simulink model "PB2M_001_007_RL"  (R2024a)
settings: Solver=FixedStepDiscrete  StartTime=0.0  StopTime=inf  FixedStep=[global_ST]  RelTol=1e-3
model workspace (MAT data in the model file):
  Var = 0
values from neighbouring files (symbols this model uses):
  global_ST = 1    [SimControl_v3_rl.m]    (also in SimControl_v4.m)
  global_time = [0:1:8784]'    [SimControl_v3_rl.m]    (also in SimControl_v4.m)
undefined symbols (not defined in the file or in its folder): acc, AEL, allActions, AMB, ATR, Bttry, CGH2, CGO2, CHP, COMPR, contActSpace, Ctrl, DiscIntNeverNeededParam, DIST, DRY, GASF, Gasf, imit_action_noise_variance, lowerLim, MES, NumEpisodes, NumImitLearning, numtraineps, PV, th, upperLim, vanilla, WT
libraries: simulink x1, rllib x1
(part 1 of 2)
settings Model: Creator=hogrebe  LastModifiedBy=salomon_p
settings SolverCC: AlgebraicLoopSolver=TrustRegion
settings DataIOCC: SaveOutput=off  DSMLogging=off  InspectSignalLogs=on  SaveTime=off
settings OptimizationCC: BlockReduction=off
settings DebuggingCC: SignalInfNanChecking=error  UnconnectedInputMsg=warning  UnconnectedOutputMsg=warning  UnconnectedLineMsg=warning
settings ModelReferenceCC: EnableRefExpFcnMdlSchedulingChecks=on
settings RTWCC: GPUComputeCapability=3.5  DLArmComputeVersion=19.05

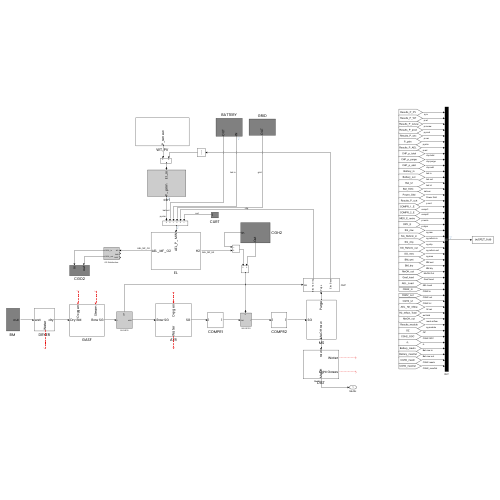
[thumbnail: Simulink's stored preview of the top-level diagram]
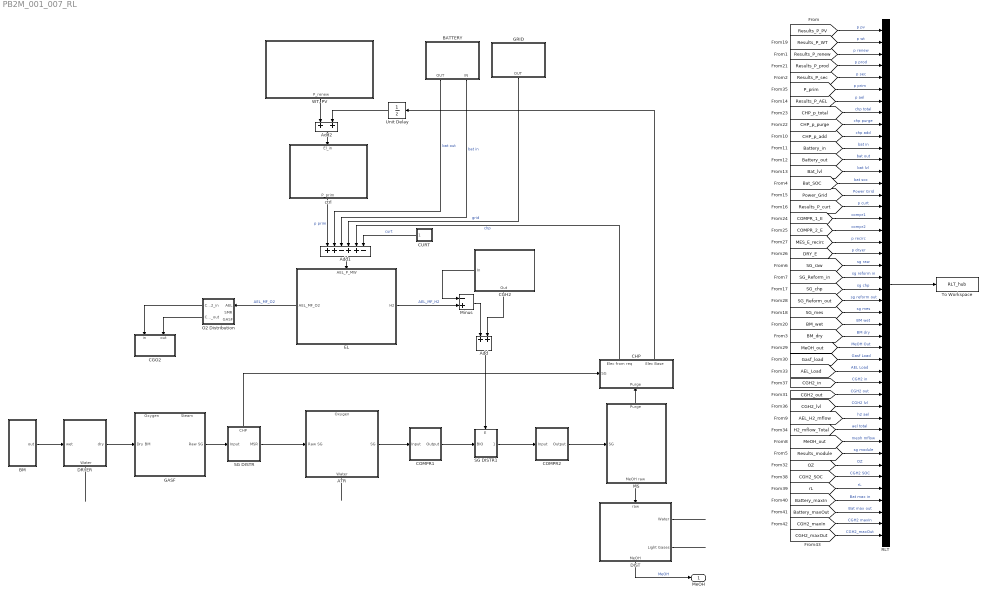
== system PB2M_001_007_RL ==
  ATR : Subsystem
      settings: PortSchema="{\"entries\":[{\"content\":{\"sides\":[{\"content\":{\"connectorIds\":[\"In1\"]},\"type\":\"ConnectorPlacement.EquallySpacedRectSide\",\"uuid\":\"d95d7370-a768-4e71-99c5-23d50f67aabe\"},{\"content\":{\"connectorIds\":[\"Out1\"],\"side\":\"RIGHT\"},\"type\":\"ConnectorPlacement.EquallySpacedRectSide\",\"uuid\":\"3437d418-ce7d-423d-8668-067a2caa5d39\"},{\"content\":{\"connectorIds\":[\"In2\"],\"side\":\"TOP\"},\"type\":\"ConnectorPlacement.EquallySpacedRectSide\",\"uuid\":\"c8aa7c63-1393-4bbc-8660-d82006d9d42e\"},{\"content\":{\"connectorIds\":[\"Out2\"],\"side\":\"BOTTOM\"},\"type\":\"ConnectorPlacement.EquallySpacedRectSide\",\"uuid\":\"8d079498-92c7-4ac5-81b3-d100ec68b2bd\"}]},\"type\":\"ConnectorPlacement.EquallySpacedConnector\",\"uuid\":\"07712eec-a256-4c23-80e6-026550a38bce\"}],\"packageUris\":[\"http://schema.mathworks.com/mf0/Connector/R2020b\"],\"version\":\"1.0\"}"
  Add : Sum
  Add1 : Sum  Inputs=++-++-
  Add2 : Sum
  BATTERY : Subsystem
      settings: PortSchema="{\"entries\":[{\"content\":{\"sides\":[{\"content\":{},\"type\":\"ConnectorPlacement.EquallySpacedRectSide\",\"uuid\":\"b156ae25-26b3-4eee-ac7f-e302bdaac2ab\"},{\"content\":{\"side\":\"RIGHT\"},\"type\":\"ConnectorPlacement.EquallySpacedRectSide\",\"uuid\":\"f3a3b929-51c5-4419-b41e-ec6279a18565\"},{\"content\":{\"side\":\"TOP\"},\"type\":\"ConnectorPlacement.EquallySpacedRectSide\",\"uuid\":\"01f6443f-63f0-4718-804f-9bad3a04ddfb\"},{\"content\":{\"connectorIds\":[\"Out1\",\"Out2\"],\"side\":\"BOTTOM\"},\"type\":\"ConnectorPlacement.EquallySpacedRectSide\",\"uuid\":\"cbf48387-64e5-4e53-bde3-6e14dbb130f7\"}]},\"type\":\"ConnectorPlacement.EquallySpacedConnector\",\"uuid\":\"4aa34124-3e08-49a0-9db9-a8367ba9f9e9\"}],\"packageUris\":[\"http://schema.mathworks.com/mf0/Connector/R2020b\"],\"version\":\"1.0\"}"
  "BM " : Subsystem
      settings: PortSchema="{\"entries\":[{\"content\":{\"sides\":[{\"content\":{},\"type\":\"ConnectorPlacement.EquallySpacedRectSide\",\"uuid\":\"b6854826-029a-462c-abc7-1ad3a9c8d91d\"},{\"content\":{\"side\":\"RIGHT\"},\"type\":\"ConnectorPlacement.EquallySpacedRectSide\",\"uuid\":\"c18fafb4-eebd-4b53-a025-0d4bc890a5f2\"},{\"content\":{\"connectorIds\":[\"Out1\"],\"side\":\"TOP\"},\"type\":\"ConnectorPlacement.EquallySpacedRectSide\",\"uuid\":\"39a115de-f541-49b1-95b5-0fdea67e1df4\"}]},\"type\":\"ConnectorPlacement.EquallySpacedConnector\",\"uuid\":\"d3505c7c-2ca5-40d6-998f-e51c69df56d8\"}],\"packageUris\":[\"http://schema.mathworks.com/mf0/Connector/R2020b\"],\"version\":\"1.0\"}"
  CGH2 : Subsystem
      settings: PortSchema="{\"entries\":[{\"content\":{\"sides\":[{\"content\":{\"connectorIds\":[\"Out2\"]},\"type\":\"ConnectorPlacement.EquallySpacedRectSide\",\"uuid\":\"c54b6fc4-3adc-4d22-bd7c-d1fb71d09cc2\"},{\"content\":{\"side\":\"RIGHT\"},\"type\":\"ConnectorPlacement.EquallySpacedRectSide\",\"uuid\":\"cb46d28f-124e-4362-a527-4ffafd6ca6aa\"},{\"content\":{\"side\":\"TOP\"},\"type\":\"ConnectorPlacement.EquallySpacedRectSide\",\"uuid\":\"cd2bfd56-c3bb-4b21-97bf-19e28abe6737\"},{\"content\":{\"connectorIds\":[\"Out1\"],\"side\":\"BOTTOM\"},\"type\":\"ConnectorPlacement.EquallySpacedRectSide\",\"uuid\":\"e393c782-34b5-435a-9a6b-fea68a5f76b1\"}]},\"type\":\"ConnectorPlacement.EquallySpacedConnector\",\"uuid\":\"04f91959-6cb0-408d-b188-ebba459e7bf2\"}],\"packageUris\":[\"http://schema.mathworks.com/mf0/Connector/R2020b\"],\"version\":\"1.0\"}"
  CGO2 : Subsystem
      settings: PortSchema="{\"entries\":[{\"content\":{\"sides\":[{\"content\":{},\"type\":\"ConnectorPlacement.EquallySpacedRectSide\",\"uuid\":\"5fd0e465-b758-40c5-99c0-bd502cf80220\"},{\"content\":{\"side\":\"RIGHT\"},\"type\":\"ConnectorPlacement.EquallySpacedRectSide\",\"uuid\":\"8c2bf71d-dd8a-4c38-9726-2100ecfb4157\"},{\"content\":{\"connectorIds\":[\"In1\",\"In2\"],\"side\":\"TOP\"},\"type\":\"ConnectorPlacement.EquallySpacedRectSide\",\"uuid\":\"9b00925e-eb9b-456e-968f-5d87047a8706\"}]},\"type\":\"ConnectorPlacement.EquallySpacedConnector\",\"uuid\":\"2f6cfec4-9fe2-41ff-9b0f-2d3a7383541d\"}],\"packageUris\":[\"http://schema.mathworks.com/mf0/Connector/R2020b\"],\"version\":\"1.0\"}"
  CHP : Subsystem
      settings: PortSchema="{\"entries\":[{\"content\":{\"sides\":[{\"content\":{\"connectorIds\":[\"In1\"]},\"type\":\"ConnectorPlacement.EquallySpacedRectSide\",\"uuid\":\"455e4cb2-b7ce-40b3-9267-45576cb92a35\"},{\"content\":{\"side\":\"RIGHT\"},\"type\":\"ConnectorPlacement.EquallySpacedRectSide\",\"uuid\":\"26266506-6e66-4bc0-bccd-a9e779dcae16\"},{\"content\":{\"connectorIds\":[\"Out1\",\"Out2\"],\"side\":\"TOP\"},\"type\":\"ConnectorPlacement.EquallySpacedRectSide\",\"uuid\":\"0bfe460e-97a8-4cdd-8918-1c56f22f3fbd\"},{\"content\":{\"connectorIds\":[\"In2\"],\"side\":\"BOTTOM\"},\"type\":\"ConnectorPlacement.EquallySpacedRectSide\",\"uuid\":\"d15a681e-1531-4d34-b913-d07bfab7e09a\"}]},\"type\":\"ConnectorPlacement.EquallySpacedConnector\",\"uuid\":\"864e4265-4fc9-4c94-8dd3-96a5c52575a2\"}],\"packageUris\":[\"http://schema.mathworks.com/mf0/Connector/R2020b\"],\"version\":\"1.0\"}"
  COMPR1 : Subsystem
  COMPR2 : Subsystem
  CURT : Subsystem
      settings: PortSchema="{\"entries\":[{\"content\":{\"sides\":[{\"content\":{\"connectorIds\":[\"Out1\"]},\"type\":\"ConnectorPlacement.EquallySpacedRectSide\",\"uuid\":\"455e4cb2-b7ce-40b3-9267-45576cb92a35\"},{\"content\":{\"side\":\"RIGHT\"},\"type\":\"ConnectorPlacement.EquallySpacedRectSide\",\"uuid\":\"26266506-6e66-4bc0-bccd-a9e779dcae16\"},{\"content\":{\"side\":\"TOP\"},\"type\":\"ConnectorPlacement.EquallySpacedRectSide\",\"uuid\":\"0bfe460e-97a8-4cdd-8918-1c56f22f3fbd\"}]},\"type\":\"ConnectorPlacement.EquallySpacedConnector\",\"uuid\":\"864e4265-4fc9-4c94-8dd3-96a5c52575a2\"}],\"packageUris\":[\"http://schema.mathworks.com/mf0/Connector/R2020b\"],\"version\":\"1.0\"}"
  DIST : Subsystem
      settings: PortSchema="{\"entries\":[{\"content\":{\"sides\":[{\"content\":{},\"type\":\"ConnectorPlacement.EquallySpacedRectSide\",\"uuid\":\"9bb20e76-c8c0-4ce3-bfa2-fd978c659bcc\"},{\"content\":{\"connectorIds\":[\"Out1\",\"Out2\"],\"side\":\"RIGHT\"},\"type\":\"ConnectorPlacement.EquallySpacedRectSide\",\"uuid\":\"12d31df4-77c9-4a5c-9a6c-fd7c89038c05\"},{\"content\":{\"connectorIds\":[\"In1\"],\"side\":\"TOP\"},\"type\":\"ConnectorPlacement.EquallySpacedRectSide\",\"uuid\":\"3a96496e-8d88-4b7f-91f0-6f8e8152b6d3\"},{\"content\":{\"connectorIds\":[\"Out3\"],\"side\":\"BOTTOM\"},\"type\":\"ConnectorPlacement.EquallySpacedRectSide\",\"uuid\":\"4bc833e2-fc0a-44a4-bcf0-3ebf0863e835\"}]},\"type\":\"ConnectorPlacement.EquallySpacedConnector\",\"uuid\":\"bb9c8f09-08c9-4a34-bdc9-5c844495fddc\"}],\"packageUris\":[\"http://schema.mathworks.com/mf0/Connector/R2020b\"],\"version\":\"1.0\"}"
  DRYER : Subsystem
      settings: PortSchema="{\"entries\":[{\"content\":{\"sides\":[{\"content\":{},\"type\":\"ConnectorPlacement.EquallySpacedRectSide\",\"uuid\":\"4ebfcccc-776f-4872-9d0b-9643b5960bad\"},{\"content\":{\"connectorIds\":[\"Out1\"],\"side\":\"RIGHT\"},\"type\":\"ConnectorPlacement.EquallySpacedRectSide\",\"uuid\":\"52af1a20-21ba-42da-ac0d-5cc3ed928415\"},{\"content\":{\"connectorIds\":[\"Out2\"],\"side\":\"TOP\"},\"type\":\"ConnectorPlacement.EquallySpacedRectSide\",\"uuid\":\"35b3f618-6f56-49d4-89a8-2314405479bc\"},{\"content\":{\"connectorIds\":[\"In1\"],\"side\":\"BOTTOM\"},\"type\":\"ConnectorPlacement.EquallySpacedRectSide\",\"uuid\":\"a7ad5d18-a31c-4405-a5bd-3fe59bb19813\"}]},\"type\":\"ConnectorPlacement.EquallySpacedConnector\",\"uuid\":\"90f717a7-269d-4abb-8032-a33661c35212\"}],\"packageUris\":[\"http://schema.mathworks.com/mf0/Connector/R2020b\"],\"version\":\"1.0\"}"
  EL : Subsystem
      settings: PortSchema="{\"entries\":[{\"content\":{\"sides\":[{\"content\":{\"connectorIds\":[\"Out2\"]},\"type\":\"ConnectorPlacement.EquallySpacedRectSide\",\"uuid\":\"e86b81d9-d45f-45ad-8c80-2ef5c9159145\"},{\"content\":{\"connectorIds\":[\"Out1\"],\"side\":\"RIGHT\"},\"type\":\"ConnectorPlacement.EquallySpacedRectSide\",\"uuid\":\"b091bd34-fe91-455d-8135-92fc1e1b5bd7\"},{\"content\":{\"connectorIds\":[\"In1\"],\"side\":\"TOP\"},\"type\":\"ConnectorPlacement.EquallySpacedRectSide\",\"uuid\":\"804c6318-ad33-4a07-b17e-e0d2fd6b4b2f\"}]},\"type\":\"ConnectorPlacement.EquallySpacedConnector\",\"uuid\":\"e581105a-7c66-468d-8489-1abddd5a4bb6\"}],\"packageUris\":[\"http://schema.mathworks.com/mf0/Connector/R2020b\"],\"version\":\"1.0\"}"
  GASF : Subsystem
      settings: PortSchema="{\"entries\":[{\"content\":{\"sides\":[{\"content\":{\"connectorIds\":[\"In1\"]},\"type\":\"ConnectorPlacement.EquallySpacedRectSide\",\"uuid\":\"5e6aa46e-d817-493b-8b8b-abb4dd1f40ec\"},{\"content\":{\"connectorIds\":[\"Out1\"],\"side\":\"RIGHT\"},\"type\":\"ConnectorPlacement.EquallySpacedRectSide\",\"uuid\":\"1936bb9e-e226-4528-9325-ecfa0f913ec2\"},{\"content\":{\"connectorIds\":[\"In2\",\"In3\"],\"side\":\"TOP\"},\"type\":\"ConnectorPlacement.EquallySpacedRectSide\",\"uuid\":\"7345e236-0dce-483e-9dbc-f4ebd743c5fa\"}]},\"type\":\"ConnectorPlacement.EquallySpacedConnector\",\"uuid\":\"c88779f2-c803-4e9a-bd9c-ad3f8fae613a\"}],\"packageUris\":[\"http://schema.mathworks.com/mf0/Connector/R2020b\"],\"version\":\"1.0\"}"
  GRID : Subsystem
      settings: PortSchema="{\"entries\":[{\"content\":{\"sides\":[{\"content\":{},\"type\":\"ConnectorPlacement.EquallySpacedRectSide\",\"uuid\":\"13ddf689-c473-4fae-8488-05ba2c53be01\"},{\"content\":{\"side\":\"RIGHT\"},\"type\":\"ConnectorPlacement.EquallySpacedRectSide\",\"uuid\":\"3edd6540-09f8-47a0-8af0-925a1a207bbe\"},{\"content\":{\"side\":\"TOP\"},\"type\":\"ConnectorPlacement.EquallySpacedRectSide\",\"uuid\":\"e7e0af70-0c4e-4701-890f-2bc2f1b60263\"},{\"content\":{\"connectorIds\":[\"Out1\"],\"side\":\"BOTTOM\"},\"type\":\"ConnectorPlacement.EquallySpacedRectSide\",\"uuid\":\"aae9c7fc-ae1b-458f-888e-dcbddd5e368f\"}]},\"type\":\"ConnectorPlacement.EquallySpacedConnector\",\"uuid\":\"9fa59c12-9be8-49ba-a862-8cdac5f592f4\"}],\"packageUris\":[\"http://schema.mathworks.com/mf0/Connector/R2020b\"],\"version\":\"1.0\"}"
  MS : Subsystem
      settings: PortSchema="{\"entries\":[{\"content\":{\"sides\":[{\"content\":{\"connectorIds\":[\"In1\"]},\"type\":\"ConnectorPlacement.EquallySpacedRectSide\",\"uuid\":\"7c68cb95-e770-413e-a40e-672fd8604812\"},{\"content\":{\"side\":\"RIGHT\"},\"type\":\"ConnectorPlacement.EquallySpacedRectSide\",\"uuid\":\"6240a65a-2dbc-4a6e-817e-2ab31946396e\"},{\"content\":{\"connectorIds\":[\"Out2\"],\"side\":\"TOP\"},\"type\":\"ConnectorPlacement.EquallySpacedRectSide\",\"uuid\":\"1a1b519e-0693-45b9-a906-950b0dca57a1\"},{\"content\":{\"connectorIds\":[\"Out1\"],\"side\":\"BOTTOM\"},\"type\":\"ConnectorPlacement.EquallySpacedRectSide\",\"uuid\":\"e87dd805-e630-4a2f-8388-2c51cd14fe9e\"}]},\"type\":\"ConnectorPlacement.EquallySpacedConnector\",\"uuid\":\"e16e5d91-de04-48fc-b44b-fdb042a92f84\"}],\"packageUris\":[\"http://schema.mathworks.com/mf0/Connector/R2020b\"],\"version\":\"1.0\"}"
  Minus : Sum  Inputs=-+
  O2 Distribution : Subsystem
      settings: PortSchema="{\"entries\":[{\"content\":{\"sides\":[{\"content\":{\"connectorIds\":[\"Out3\",\"Out4\"]},\"type\":\"ConnectorPlacement.EquallySpacedRectSide\",\"uuid\":\"30156f9c-db5e-4257-aeed-83f2c1c2e5bf\"},{\"content\":{\"connectorIds\":[\"In1\",\"Out1\",\"Out2\"],\"side\":\"RIGHT\"},\"type\":\"ConnectorPlacement.EquallySpacedRectSide\",\"uuid\":\"c3a4c4df-5b27-475f-87a9-b45da9a3b436\"},{\"content\":{\"side\":\"TOP\"},\"type\":\"ConnectorPlacement.EquallySpacedRectSide\",\"uuid\":\"5997053d-e240-46ef-b6d7-4f9a3a1c0d15\"}]},\"type\":\"ConnectorPlacement.EquallySpacedConnector\",\"uuid\":\"10d495fb-251b-444d-bd0a-f6bbcb16daf1\"}],\"packageUris\":[\"http://schema.mathworks.com/mf0/Connector/R2020b\"],\"version\":\"1.0\"}"
  RLT : BusCreator  Inputs=44
  SG DISTR : Subsystem
      settings: PortSchema="{\"entries\":[{\"content\":{\"sides\":[{\"content\":{},\"type\":\"ConnectorPlacement.EquallySpacedRectSide\",\"uuid\":\"e86b81d9-d45f-45ad-8c80-2ef5c9159145\"},{\"content\":{\"connectorIds\":[\"Out1\"],\"side\":\"RIGHT\"},\"type\":\"ConnectorPlacement.EquallySpacedRectSide\",\"uuid\":\"b091bd34-fe91-455d-8135-92fc1e1b5bd7\"},{\"content\":{\"connectorIds\":[\"In1\"],\"side\":\"TOP\"},\"type\":\"ConnectorPlacement.EquallySpacedRectSide\",\"uuid\":\"804c6318-ad33-4a07-b17e-e0d2fd6b4b2f\"},{\"content\":{\"connectorIds\":[\"Out2\"],\"side\":\"BOTTOM\"},\"type\":\"ConnectorPlacement.EquallySpacedRectSide\",\"uuid\":\"fb2b571c-70ad-41c0-9018-552f5e98e285\"}]},\"type\":\"ConnectorPlacement.EquallySpacedConnector\",\"uuid\":\"e581105a-7c66-468d-8489-1abddd5a4bb6\"}],\"packageUris\":[\"http://schema.mathworks.com/mf0/Connector/R2020b\"],\"version\":\"1.0\"}"
  SG DISTR1 : Subsystem
      settings: PortSchema="{\"entries\":[{\"content\":{\"sides\":[{\"content\":{},\"type\":\"ConnectorPlacement.EquallySpacedRectSide\",\"uuid\":\"e9c91cab-8c69-4152-b789-7325d2e32e4b\"},{\"content\":{\"connectorIds\":[\"In2\"],\"side\":\"RIGHT\"},\"type\":\"ConnectorPlacement.EquallySpacedRectSide\",\"uuid\":\"b801369b-5c93-4438-bd90-0992b326086c\"},{\"content\":{\"connectorIds\":[\"In1\"],\"side\":\"TOP\"},\"type\":\"ConnectorPlacement.EquallySpacedRectSide\",\"uuid\":\"e103e961-9a42-4e45-906c-e9068e5e276c\"},{\"content\":{\"connectorIds\":[\"Out1\"],\"side\":\"BOTTOM\"},\"type\":\"ConnectorPlacement.EquallySpacedRectSide\",\"uuid\":\"0e96afff-5922-401c-b36e-06eb0842909a\"}]},\"type\":\"ConnectorPlacement.EquallySpacedConnector\",\"uuid\":\"2ea93f77-6b27-4245-9c93-a72fb1fe7fa6\"}],\"packageUris\":[\"http://schema.mathworks.com/mf0/Connector/R2020b\"],\"version\":\"1.0\"}"
  To Workspace : ToWorkspace  VariableName=RLT_hub  SampleTime=-1
  Unit Delay : UnitDelay  SampleTime=-1  HasFrameUpgradeWarning=on
  "WT, PV" : Subsystem
      settings: PortSchema="{\"entries\":[{\"content\":{\"sides\":[{\"content\":{},\"type\":\"ConnectorPlacement.EquallySpacedRectSide\",\"uuid\":\"8a2d1ae0-dccb-4b14-8547-5eeedb1731af\"},{\"content\":{\"side\":\"RIGHT\"},\"type\":\"ConnectorPlacement.EquallySpacedRectSide\",\"uuid\":\"3fb157a2-f839-4f36-8a45-db822d022818\"},{\"content\":{\"side\":\"TOP\"},\"type\":\"ConnectorPlacement.EquallySpacedRectSide\",\"uuid\":\"528eda02-61b1-46fc-814d-d4347d4497c7\"},{\"content\":{\"connectorIds\":[\"Out1\"],\"side\":\"BOTTOM\"},\"type\":\"ConnectorPlacement.EquallySpacedRectSide\",\"uuid\":\"9515b46c-adb3-49ca-b783-afbfd8bcb61a\"}]},\"type\":\"ConnectorPlacement.EquallySpacedConnector\",\"uuid\":\"11973188-1db2-4f1c-be62-25a3f427210a\"}],\"packageUris\":[\"http://schema.mathworks.com/mf0/Connector/R2020b\"],\"version\":\"1.0\"}"
  ctrl : Subsystem
      settings: PortSchema="{\"entries\":[{\"content\":{\"sides\":[{\"content\":{},\"type\":\"ConnectorPlacement.EquallySpacedRectSide\",\"uuid\":\"29211eeb-3776-4ac1-8b6e-260e730243bf\"},{\"content\":{\"side\":\"RIGHT\"},\"type\":\"ConnectorPlacement.EquallySpacedRectSide\",\"uuid\":\"53fb8f12-056e-46ec-aa17-61752852cd78\"},{\"content\":{\"connectorIds\":[\"In1\"],\"side\":\"TOP\"},\"type\":\"ConnectorPlacement.EquallySpacedRectSide\",\"uuid\":\"01e66cb5-7d7a-44e4-93db-ae92dadb6fda\"},{\"content\":{\"connectorIds\":[\"Out1\"],\"side\":\"BOTTOM\"},\"type\":\"ConnectorPlacement.EquallySpacedRectSide\",\"uuid\":\"c79a4ef3-496c-4d69-ab69-9c29ac94c10a\"}]},\"type\":\"ConnectorPlacement.EquallySpacedConnector\",\"uuid\":\"562cb731-47de-4bfb-9a4e-cc780a8c656b\"}],\"packageUris\":[\"http://schema.mathworks.com/mf0/Connector/R2020b\"],\"version\":\"1.0\"}"
  MeOH : Outport
  wires:
  EL/2(AEL_MF_O2) -> O2 Distribution/1(AEL)  "AEL_MF_O2"
  O2 Distribution/4(CGO2_out) -> CGO2/2(out)
  O2 Distribution/3(CGO2_in) -> CGO2/1(in)
  SG DISTR/2(MSR) -> ATR/1(Raw SG)
  DRYER/2(dry) -> GASF/1(Dry BM)
  GASF/1(Raw SG) -> SG DISTR/1(Input)
  ATR/1(SG) -> COMPR1/1(Input)
  SG DISTR1/1(Output) -> COMPR2/1(Input)
  SG DISTR/1(CHP) -> CHP/1(SG)
  "BM "/1(out) -> DRYER/1(wet)
  COMPR2/1(Output) -> MS/1(SG)
  ctrl/1(P_prim) -> Add1/1  "p prim"
  Add1/1 -> EL/1(AEL_P_MW)
  CHP/1(Elec from req) -> Add1/5  "chp"
  BATTERY/1(OUT) -> Add1/2  "bat out"
  BATTERY/2(IN) -> Add1/3  "bat in"
  GRID/1(OUT) -> Add1/4  "grid"
  CURT/1(Output) -> Add1/6  "curt"
  COMPR1/1(Output) -> SG DISTR1/1(BIO)
  RLT/1 -> To Workspace/1
  [SG_raw] -> RLT/21  "sg raw"
  [COMPR_2_E] -> RLT/18  "compr2"
  [Results_P_PV] -> RLT/1  "p pv"
  [Results_P_renew] -> RLT/3  "p renew"
  [Results_P_curt] -> RLT/16  "p curt"
  [Battery_in] -> RLT/11  "bat in"
  [Power_Grid] -> RLT/15  "Power Grid"
  [Bat_SOC] -> RLT/14  "bat soc"
  [CHP_p_purge] -> RLT/9  "chp purge"
  [Results_P_AEL] -> RLT/7  "p ael"
  [P_prim] -> RLT/6  "p prim"
  [CHP_p_total] -> RLT/8  "chp total"
  [COMPR_1_E] -> RLT/17  "compr1"
  [Results_P_sec] -> RLT/5  "p sec"
  [MES_E_recirc] -> RLT/19  "p recirc"
  MS/2(Purge) -> CHP/2(Purge)
  Add2/1 -> ctrl/1(El_in)
  "WT, PV"/1(P_renew) -> Add2/1
  DRYER/1(Water) -> ?
  ATR/2(Water) -> ?
  MS/1(MeOH raw) -> DIST/1(raw)
  DIST/3(MeOH) -> MeOH/1  "MeOH"
  DIST/1(Water) -> ?
  DIST/2(Light Gases) -> ?
  [SG_Reform_in] -> RLT/22  "sg reform in"
  [Results_P_prod] -> RLT/4  "p prod"
  [Battery_out] -> RLT/12  "bat out"
  [Bat_lvl] -> RLT/13  "bat lvl"
  [Results_P_WT] -> RLT/2  "p wt"
  ? -> GASF/3(Steam)
  ? -> GASF/2(Oxygen)
  ? -> ATR/2(Oxygen)
  [SG_Reform_out] -> RLT/24  "sg reform out"
  [SG_mes] -> RLT/25  "sg mes"
  [BM_wet] -> RLT/26  "BM wet"
  [BM_dry] -> RLT/27  "BM dry"
  [MeOH_out] -> RLT/28  "MeOH Out"
  CHP/2(Elec Base) -> Unit Delay/1
  Unit Delay/1 -> Add2/2
  CGH2/1(Out) -> Add/2
  [Gasf_load] -> RLT/29  "Gasf Load"
  [CGH2_in] -> RLT/31  "CGH2 in"
  EL/1(H2) -> Minus/2  "AEL_MF_H2"
  Minus/1 -> Add/1
  CGH2/2(In) -> Minus/1
  [H2_mflow_Total] -> RLT/35  "ael total"
  [CHP_p_add] -> RLT/10  "chp add"
  [SG_chp] -> RLT/23  "sg chp"
  [DRY_E] -> RLT/20  "p dryer"
  [AEL_Load] -> RLT/30  "AEL Load"
  [CGH2_out] -> RLT/32  "CGH2 out"
  [CGH2_lvl] -> RLT/33  "CGH2 lvl"
  [AEL_H2_mflow] -> RLT/34  "h2 ael"
  [MeOH_out] -> RLT/36  "meoh mflow"
  [Results_module] -> RLT/37  "sg module"
  [OZ] -> RLT/38  "OZ"
  Add/1 -> SG DISTR1/2(E)
  [CGH2_SOC] -> RLT/39  "CGH2 SOC"
  [rL] -> RLT/40  "rL"
  [Battery_maxIn] -> RLT/41  "Bat max in"
  [Battery_maxOut] -> RLT/42  "Bat max out"
  [CGH2_maxIn] -> RLT/43  "CGH2 maxIn"
  [CGH2_maxOut] -> RLT/44  "CGH2_maxOut"

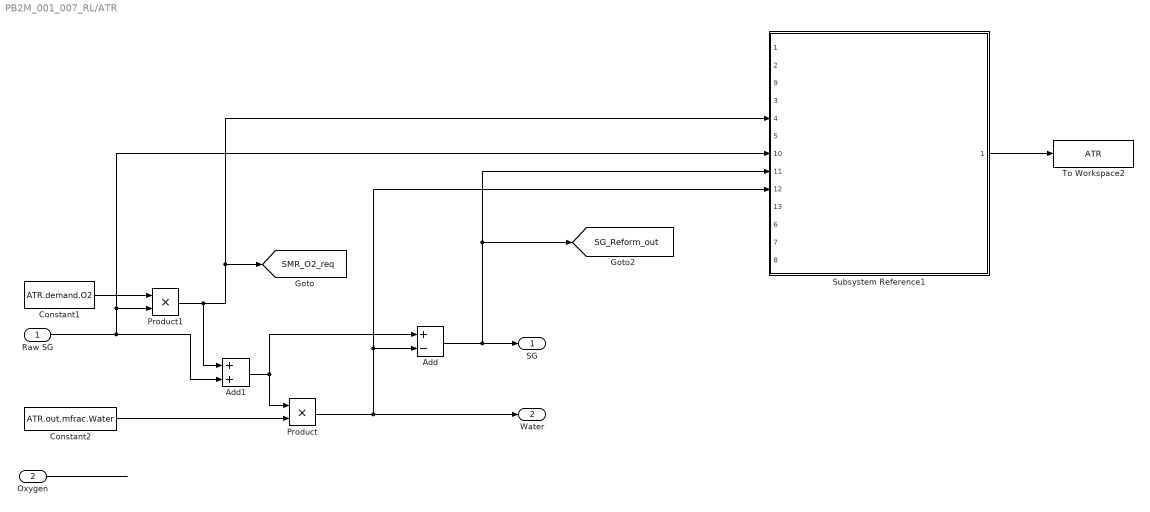
== system PB2M_001_007_RL/ATR ==
  Raw SG : Inport
  Oxygen : Inport  Port=2
  Add : Sum  Inputs=+-
  Add1 : Sum
  Constant1 : Constant  Value=ATR.demand.O2
  Constant2 : Constant  Value=ATR.out.mfrac.Water
  Product : Product
  Product1 : Product
  Subsystem Reference1 : Subsystem  ReferencedSubsystem=PB2M_RltHub_002
      settings: PortSchema="{\"entries\":[{\"content\":{\"sides\":[{\"content\":{\"connectorIds\":[\"In1\",\"In2\",\"In9\",\"In3\",\"In4\",\"In5\",\"In10\",\"In11\",\"In12\",\"In13\",\"In6\",\"In7\",\"In8\"]},\"type\":\"ConnectorPlacement.EquallySpacedRectSide\",\"uuid\":\"c0facf1f-1082-4e5e-a2dc-e6e5892eaa43\"},{\"content\":{\"connectorIds\":[\"Out1\"],\"side\":\"RIGHT\"},\"type\":\"ConnectorPlacement.EquallySpacedRectSide\",\"uuid\":\"0b7dd7b0-e6ba-4d46-903a-281e0aa5a817\"},{\"content\":{\"side\":\"TOP\"},\"type\":\"ConnectorPlacement.EquallySpacedRectSide\",\"uuid\":\"7e96b7db-a9f3-428f-bb56-8b966044c518\"}]},\"type\":\"ConnectorPlacement.EquallySpacedConnector\",\"uuid\":\"c0112396-a54d-4537-ae03-3d933c26b43e\"}],\"packageUris\":[\"http://schema.mathworks.com/mf0/Connector/R2020b\"],\"version\":\"1.0\"}"
  To Workspace2 : ToWorkspace  VariableName=ATR  SampleTime=-1
  SG : Outport
  Water : Outport  Port=2
  tag scope: SG_Reform_out=global, SMR_O2_req=global
  wires:
  Product1/1 -> [SMR_O2_req], Subsystem Reference1/4, Add1/1
  Raw SG/1 -> Product1/2, Subsystem Reference1/10, Add1/2
  Constant2/1 -> Product/2
  Product/1 -> Water/1, Subsystem Reference1/12, Add/2
  Add/1 -> [SG_Reform_out], Subsystem Reference1/11, SG/1
  Oxygen/1 -> ?
  Subsystem Reference1/1 -> To Workspace2/1
  Constant1/1 -> Product1/1
  Add1/1 -> Add/1, Product/1

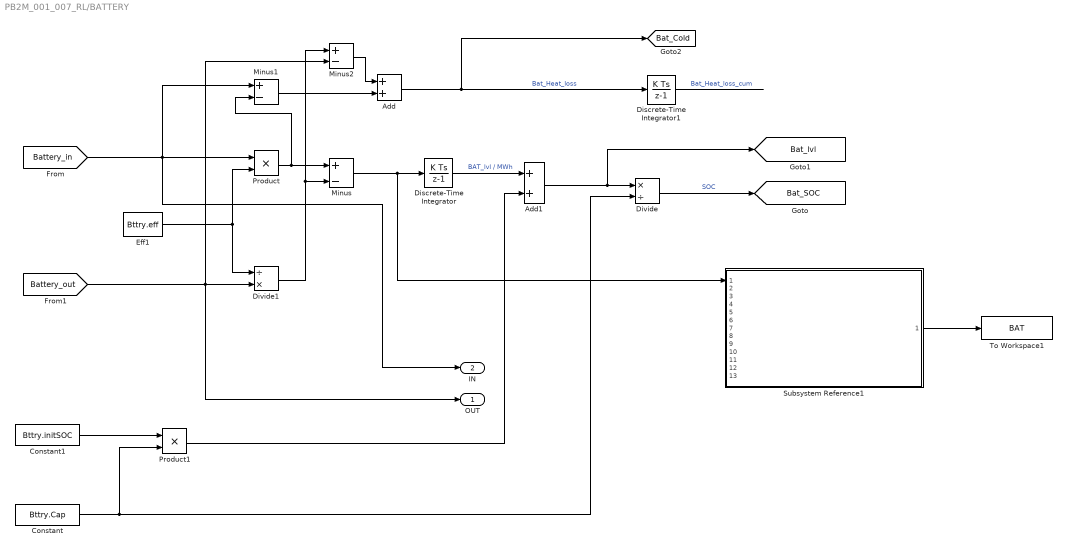
== system PB2M_001_007_RL/BATTERY ==
  Add : Sum
  Add1 : Sum
  Constant : Constant  Value=Bttry.Cap
  Constant1 : Constant  Value=Bttry.initSOC
  Discrete-Time Integrator : DiscreteIntegrator  SampleTime=-1  ICPrevOutput=DiscIntNeverNeededParam  ICPrevScaledInput=DiscIntNeverNeededParam
  Discrete-Time Integrator1 : DiscreteIntegrator  SampleTime=-1  ICPrevOutput=DiscIntNeverNeededParam  ICPrevScaledInput=DiscIntNeverNeededParam
  Divide : Product  Inputs=*/
  Divide1 : Product  Inputs=/*
  Eff1 : Constant  Value=Bttry.eff
  Minus : Sum  Inputs=+-
  Minus1 : Sum  Inputs=+-
  Minus2 : Sum  Inputs=+-
  Product : Product
  Product1 : Product
  Subsystem Reference1 : Subsystem  ReferencedSubsystem=PB2M_RltHub_002
  To Workspace1 : ToWorkspace  VariableName=BAT  SampleTime=-1
  OUT : Outport
  IN : Outport  Port=2
  tag scope: Bat_Cold=global, Bat_SOC=global, Bat_lvl=global
  wires:
  Constant/1 -> Divide/2, Product1/2
  Divide/1 -> [Bat_SOC]  "SOC"
  Product/1 -> Minus1/2, Minus/1
  Divide1/1 -> Minus2/1, Minus/2
  Eff1/1 -> Divide1/1, Product/2
  Minus1/1 -> Add/2
  Minus2/1 -> Add/1
  Add/1 -> [Bat_Cold], Discrete-Time Integrator1/1  "Bat_Heat_loss"
  Discrete-Time Integrator1/1 -> ?  "Bat_Heat_loss_cum"
  [Battery_out] -> Divide1/2, OUT/1, Minus2/2
  [Battery_in] -> IN/1, Minus1/1, Product/1
  Minus/1 -> Subsystem Reference1/1, Discrete-Time Integrator/1
  Add1/1 -> [Bat_lvl], Divide/1
  Discrete-Time Integrator/1 -> Add1/1  "BAT_lvl / MWh"
  Product1/1 -> Add1/2
  Subsystem Reference1/1 -> To Workspace1/1
  Constant1/1 -> Product1/1

== system PB2M_001_007_RL/BM  ==
  Constant1 : Constant  Value=10.1
  IC : InitialCondition
  Ideal Controller : MATLAB Function  TreatAsAtomicUnit=on
  MATLAB Function : MATLAB Function  TreatAsAtomicUnit=on
  Subsystem Reference1 : Subsystem  ReferencedSubsystem=PB2M_RltHub_002
  To Workspace1 : ToWorkspace  VariableName=BM  SampleTime=-1
  out : Outport
  tag scope: BM_wet=global, Results_module=global
  wires:
  MATLAB Function/1(module) -> IC/1  "module"
  [H2_mflow_Total] -> Ideal Controller/3(Hydrogen), MATLAB Function/1(mflow_H2)  "H2 total"
  [SG_Reform_out] -> MATLAB Function/2(mflow_SG)  "sg reform out"
  IC/1 -> [Results_module]
  [CHP_SG_req] -> Ideal Controller/2(CHP)
  Constant1/1 -> Ideal Controller/1(fac)
  Subsystem Reference1/1 -> To Workspace1/1
  Ideal Controller/1(BM_wet) -> out/1, Subsystem Reference1/5, [BM_wet]

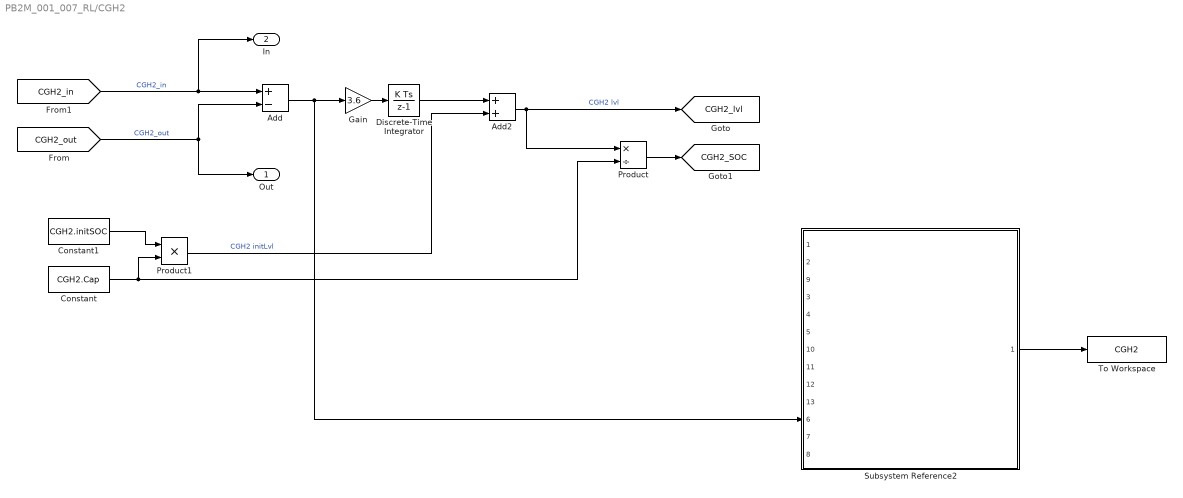
== system PB2M_001_007_RL/CGH2 ==
  Add : Sum  Inputs=+-
  Add2 : Sum
  Constant : Constant  Value=CGH2.Cap
  Constant1 : Constant  Value=CGH2.initSOC
  Discrete-Time Integrator : DiscreteIntegrator  SampleTime=-1  ICPrevOutput=DiscIntNeverNeededParam  ICPrevScaledInput=DiscIntNeverNeededParam
  Gain : Gain  Gain=3.6
  Product : Product  Inputs=*/
  Product1 : Product
  Subsystem Reference2 : Subsystem  ReferencedSubsystem=PB2M_RltHub_002
      settings: PortSchema="{\"entries\":[{\"content\":{\"sides\":[{\"content\":{\"connectorIds\":[\"In1\",\"In2\",\"In9\",\"In3\",\"In4\",\"In5\",\"In10\",\"In11\",\"In12\",\"In13\",\"In6\",\"In7\",\"In8\"]},\"type\":\"ConnectorPlacement.EquallySpacedRectSide\",\"uuid\":\"c0facf1f-1082-4e5e-a2dc-e6e5892eaa43\"},{\"content\":{\"connectorIds\":[\"Out1\"],\"side\":\"RIGHT\"},\"type\":\"ConnectorPlacement.EquallySpacedRectSide\",\"uuid\":\"0b7dd7b0-e6ba-4d46-903a-281e0aa5a817\"},{\"content\":{\"side\":\"TOP\"},\"type\":\"ConnectorPlacement.EquallySpacedRectSide\",\"uuid\":\"7e96b7db-a9f3-428f-bb56-8b966044c518\"}]},\"type\":\"ConnectorPlacement.EquallySpacedConnector\",\"uuid\":\"c0112396-a54d-4537-ae03-3d933c26b43e\"}],\"packageUris\":[\"http://schema.mathworks.com/mf0/Connector/R2020b\"],\"version\":\"1.0\"}"
  To Workspace : ToWorkspace  VariableName=CGH2  SampleTime=-1
  Out : Outport
  In : Outport  Port=2
  tag scope: CGH2_SOC=global, CGH2_lvl=global
  wires:
  [CGH2_out] -> Add/2, Out/1  "CGH2_out"
  Gain/1 -> Discrete-Time Integrator/1
  Add/1 -> Subsystem Reference2/6, Gain/1
  [CGH2_in] -> In/1, Add/1  "CGH2_in"
  Constant/1 -> Product1/2, Product/2
  Discrete-Time Integrator/1 -> Add2/1
  Subsystem Reference2/1 -> To Workspace/1
  Constant1/1 -> Product1/1
  Product1/1 -> Add2/2  "CGH2 initLvl"
  Product/1 -> [CGH2_SOC]
  Add2/1 -> Product/1, [CGH2_lvl]  "CGH2 lvl"

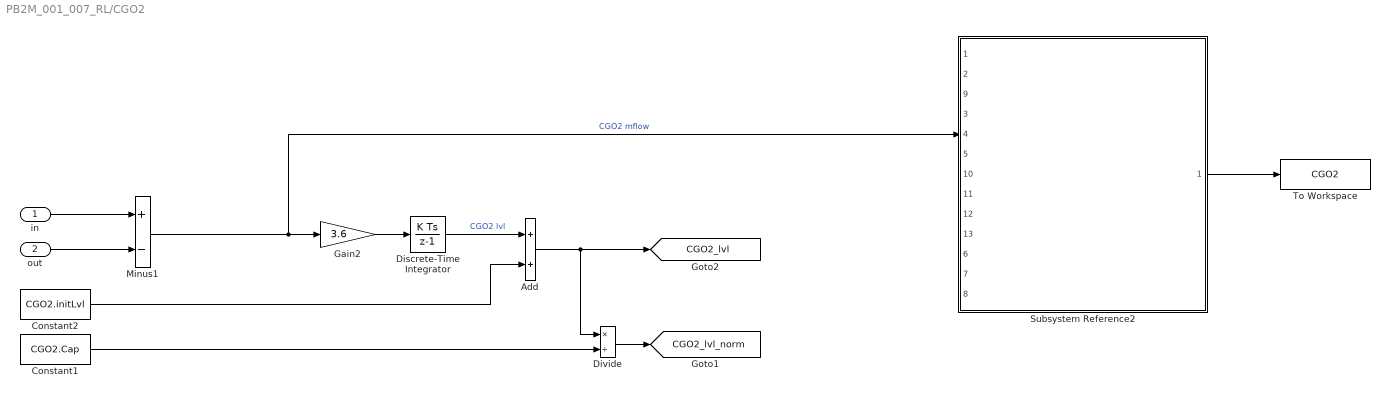
== system PB2M_001_007_RL/CGO2 ==
  in : Inport
  out : Inport  Port=2
  Add : Sum
  Constant1 : Constant  Value=CGO2.Cap
  Constant2 : Constant  Value=CGO2.initLvl
  Discrete-Time Integrator : DiscreteIntegrator  SampleTime=-1  ICPrevOutput=DiscIntNeverNeededParam  ICPrevScaledInput=DiscIntNeverNeededParam
  Divide : Product  Inputs=*/
  Gain2 : Gain  Gain=3.6
  Minus1 : Sum  Inputs=+-
  Subsystem Reference2 : Subsystem  ReferencedSubsystem=PB2M_RltHub_002
      settings: PortSchema="{\"entries\":[{\"content\":{\"sides\":[{\"content\":{\"connectorIds\":[\"In1\",\"In2\",\"In9\",\"In3\",\"In4\",\"In5\",\"In10\",\"In11\",\"In12\",\"In13\",\"In6\",\"In7\",\"In8\"]},\"type\":\"ConnectorPlacement.EquallySpacedRectSide\",\"uuid\":\"c0facf1f-1082-4e5e-a2dc-e6e5892eaa43\"},{\"content\":{\"connectorIds\":[\"Out1\"],\"side\":\"RIGHT\"},\"type\":\"ConnectorPlacement.EquallySpacedRectSide\",\"uuid\":\"0b7dd7b0-e6ba-4d46-903a-281e0aa5a817\"},{\"content\":{\"side\":\"TOP\"},\"type\":\"ConnectorPlacement.EquallySpacedRectSide\",\"uuid\":\"7e96b7db-a9f3-428f-bb56-8b966044c518\"}]},\"type\":\"ConnectorPlacement.EquallySpacedConnector\",\"uuid\":\"c0112396-a54d-4537-ae03-3d933c26b43e\"}],\"packageUris\":[\"http://schema.mathworks.com/mf0/Connector/R2020b\"],\"version\":\"1.0\"}"
  To Workspace : ToWorkspace  VariableName=CGO2  SampleTime=-1
  tag scope: CGO2_lvl=global, CGO2_lvl_norm=global
  wires:
  in/1 -> Minus1/1
  out/1 -> Minus1/2
  Minus1/1 -> Subsystem Reference2/4, Gain2/1  "CGO2 mflow"
  Gain2/1 -> Discrete-Time Integrator/1
  Discrete-Time Integrator/1 -> Add/1  "CGO2 lvl"
  Constant2/1 -> Add/2
  Add/1 -> Divide/1, [CGO2_lvl]
  Constant1/1 -> Divide/2
  Divide/1 -> [CGO2_lvl_norm]
  Subsystem Reference2/1 -> To Workspace/1

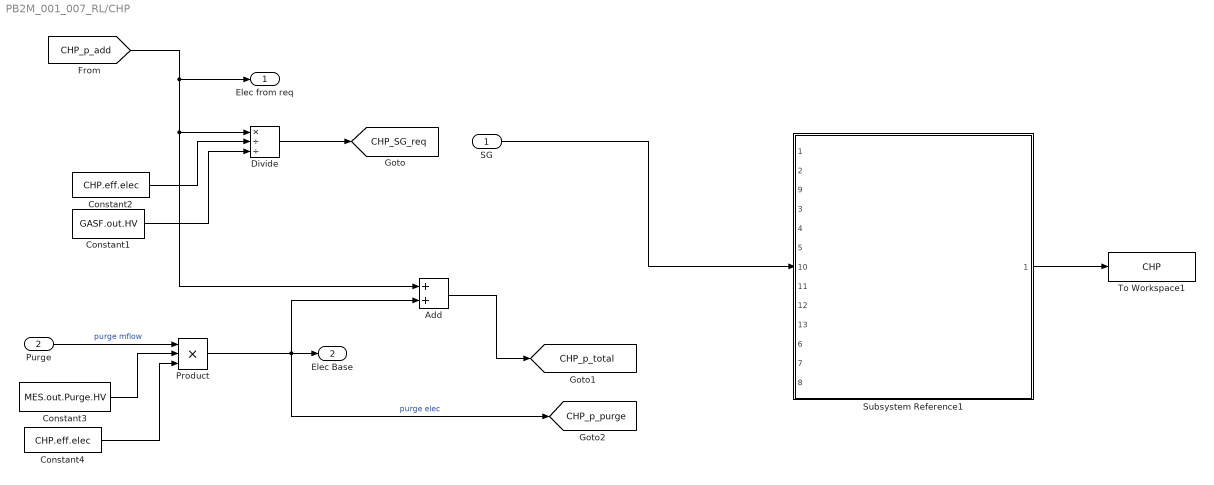
== system PB2M_001_007_RL/CHP ==
  SG : Inport
  Purge : Inport  Port=2
  Add : Sum
  Constant1 : Constant  Value=GASF.out.HV
  Constant2 : Constant  Value=CHP.eff.elec
  Constant3 : Constant  Value=MES.out.Purge.HV
  Constant4 : Constant  Value=CHP.eff.elec
  Divide : Product  Inputs=*//
  Product : Product  Inputs=***
  Subsystem Reference1 : Subsystem  ReferencedSubsystem=PB2M_RltHub_002
      settings: PortSchema="{\"entries\":[{\"content\":{\"sides\":[{\"content\":{\"connectorIds\":[\"In1\",\"In2\",\"In9\",\"In3\",\"In4\",\"In5\",\"In10\",\"In11\",\"In12\",\"In13\",\"In6\",\"In7\",\"In8\"]},\"type\":\"ConnectorPlacement.EquallySpacedRectSide\",\"uuid\":\"c0facf1f-1082-4e5e-a2dc-e6e5892eaa43\"},{\"content\":{\"connectorIds\":[\"Out1\"],\"side\":\"RIGHT\"},\"type\":\"ConnectorPlacement.EquallySpacedRectSide\",\"uuid\":\"0b7dd7b0-e6ba-4d46-903a-281e0aa5a817\"},{\"content\":{\"side\":\"TOP\"},\"type\":\"ConnectorPlacement.EquallySpacedRectSide\",\"uuid\":\"7e96b7db-a9f3-428f-bb56-8b966044c518\"}]},\"type\":\"ConnectorPlacement.EquallySpacedConnector\",\"uuid\":\"c0112396-a54d-4537-ae03-3d933c26b43e\"}],\"packageUris\":[\"http://schema.mathworks.com/mf0/Connector/R2020b\"],\"version\":\"1.0\"}"
  To Workspace1 : ToWorkspace  VariableName=CHP  SampleTime=-1
  Elec from req : Outport
  Elec Base : Outport  Port=2
  tag scope: CHP_SG_req=global, CHP_p_purge=global, CHP_p_total=global
  wires:
  Divide/1 -> [CHP_SG_req]
  [CHP_p_add] -> Add/1, Divide/1, Elec from req/1
  Constant2/1 -> Divide/2
  Constant1/1 -> Divide/3
  Purge/1 -> Product/1  "purge mflow"
  Constant3/1 -> Product/2
  Constant4/1 -> Product/3
  Product/1 -> [CHP_p_purge], Elec Base/1, Add/2  "purge elec"
  Add/1 -> [CHP_p_total]
  Subsystem Reference1/1 -> To Workspace1/1
  SG/1 -> Subsystem Reference1/10

== system PB2M_001_007_RL/COMPR1 ==
  Input : Inport
  Constant : Constant  Value=COMPR.SG.E_spec
  Product : Product
  Subsystem Reference1 : Subsystem  ReferencedSubsystem=PB2M_RltHub_002
      settings: PortSchema="{\"entries\":[{\"content\":{\"sides\":[{\"content\":{\"connectorIds\":[\"In1\",\"In2\",\"In9\",\"In3\",\"In4\",\"In5\",\"In10\",\"In11\",\"In12\",\"In13\",\"In6\",\"In7\",\"In8\"]},\"type\":\"ConnectorPlacement.EquallySpacedRectSide\",\"uuid\":\"c0facf1f-1082-4e5e-a2dc-e6e5892eaa43\"},{\"content\":{\"connectorIds\":[\"Out1\"],\"side\":\"RIGHT\"},\"type\":\"ConnectorPlacement.EquallySpacedRectSide\",\"uuid\":\"0b7dd7b0-e6ba-4d46-903a-281e0aa5a817\"},{\"content\":{\"side\":\"TOP\"},\"type\":\"ConnectorPlacement.EquallySpacedRectSide\",\"uuid\":\"7e96b7db-a9f3-428f-bb56-8b966044c518\"}]},\"type\":\"ConnectorPlacement.EquallySpacedConnector\",\"uuid\":\"c0112396-a54d-4537-ae03-3d933c26b43e\"}],\"packageUris\":[\"http://schema.mathworks.com/mf0/Connector/R2020b\"],\"version\":\"1.0\"}"
  To Workspace2 : ToWorkspace  VariableName=COMPR1  SampleTime=-1
  Output : Outport
  tag scope: COMPR_1_E=global
  wires:
  Constant/1 -> Product/1
  Input/1 -> Product/2, Output/1
  Product/1 -> Subsystem Reference1/1, [COMPR_1_E]
  Subsystem Reference1/1 -> To Workspace2/1

== system PB2M_001_007_RL/COMPR2 ==
  Input : Inport
  Constant : Constant  Value=COMPR.MIX.E_spec
  Product : Product
  Subsystem Reference2 : Subsystem  ReferencedSubsystem=PB2M_RltHub_002
      settings: PortSchema="{\"entries\":[{\"content\":{\"sides\":[{\"content\":{\"connectorIds\":[\"In1\",\"In2\",\"In9\",\"In3\",\"In4\",\"In5\",\"In10\",\"In11\",\"In12\",\"In13\",\"In6\",\"In7\",\"In8\"]},\"type\":\"ConnectorPlacement.EquallySpacedRectSide\",\"uuid\":\"c0facf1f-1082-4e5e-a2dc-e6e5892eaa43\"},{\"content\":{\"connectorIds\":[\"Out1\"],\"side\":\"RIGHT\"},\"type\":\"ConnectorPlacement.EquallySpacedRectSide\",\"uuid\":\"0b7dd7b0-e6ba-4d46-903a-281e0aa5a817\"},{\"content\":{\"side\":\"TOP\"},\"type\":\"ConnectorPlacement.EquallySpacedRectSide\",\"uuid\":\"7e96b7db-a9f3-428f-bb56-8b966044c518\"}]},\"type\":\"ConnectorPlacement.EquallySpacedConnector\",\"uuid\":\"c0112396-a54d-4537-ae03-3d933c26b43e\"}],\"packageUris\":[\"http://schema.mathworks.com/mf0/Connector/R2020b\"],\"version\":\"1.0\"}"
  To Workspace2 : ToWorkspace  VariableName=COMPR2  SampleTime=-1
  Output : Outport
  tag scope: COMPR_2_E=global
  wires:
  Constant/1 -> Product/1
  Input/1 -> Output/1, Product/2
  Product/1 -> Subsystem Reference2/1, [COMPR_2_E]
  Subsystem Reference2/1 -> To Workspace2/1

== system PB2M_001_007_RL/CURT ==
  Output : Outport
  wires:
  [Results_P_curt] -> Output/1

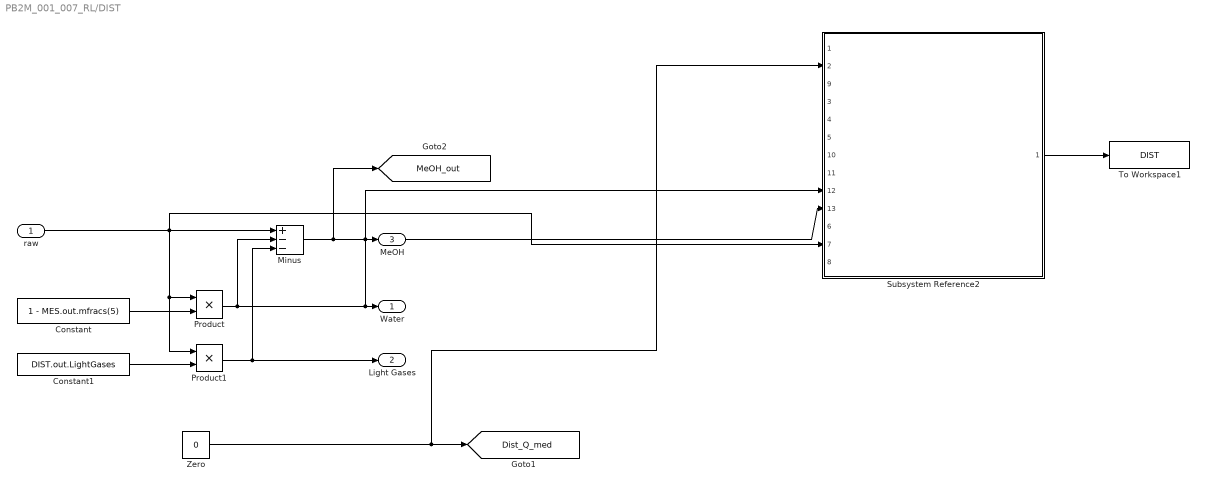
== system PB2M_001_007_RL/DIST ==
  raw : Inport
  Constant : Constant  Value=1 - MES.out.mfracs(5)
  Constant1 : Constant  Value=DIST.out.LightGases
  Minus : Sum  Inputs=+--
  Product : Product
  Product1 : Product
  Subsystem Reference2 : Subsystem  ReferencedSubsystem=PB2M_RltHub_002
      settings: PortSchema="{\"entries\":[{\"content\":{\"sides\":[{\"content\":{\"connectorIds\":[\"In1\",\"In2\",\"In9\",\"In3\",\"In4\",\"In5\",\"In10\",\"In11\",\"In12\",\"In13\",\"In6\",\"In7\",\"In8\"]},\"type\":\"ConnectorPlacement.EquallySpacedRectSide\",\"uuid\":\"c0facf1f-1082-4e5e-a2dc-e6e5892eaa43\"},{\"content\":{\"connectorIds\":[\"Out1\"],\"side\":\"RIGHT\"},\"type\":\"ConnectorPlacement.EquallySpacedRectSide\",\"uuid\":\"0b7dd7b0-e6ba-4d46-903a-281e0aa5a817\"},{\"content\":{\"side\":\"TOP\"},\"type\":\"ConnectorPlacement.EquallySpacedRectSide\",\"uuid\":\"7e96b7db-a9f3-428f-bb56-8b966044c518\"}]},\"type\":\"ConnectorPlacement.EquallySpacedConnector\",\"uuid\":\"c0112396-a54d-4537-ae03-3d933c26b43e\"}],\"packageUris\":[\"http://schema.mathworks.com/mf0/Connector/R2020b\"],\"version\":\"1.0\"}"
  To Workspace1 : ToWorkspace  VariableName=DIST  SampleTime=-1
  Zero : Constant  Value=0  OutDataTypeStr=Inherit: Inherit via back propagation
  Water : Outport
  Light Gases : Outport  Port=2
  MeOH : Outport  Port=3
  tag scope: Dist_Q_med=global, MeOH_out=global
  wires:
  Zero/1 -> [Dist_Q_med], Subsystem Reference2/2
  raw/1 -> Product/1, Product1/1, Minus/1, Subsystem Reference2/7
  Constant/1 -> Product/2
  Product/1 -> Subsystem Reference2/12, Water/1, Minus/2
  Constant1/1 -> Product1/2
  Product1/1 -> Light Gases/1, Minus/3
  Subsystem Reference2/1 -> To Workspace1/1
  Minus/1 -> Subsystem Reference2/13, MeOH/1, [MeOH_out]

== system PB2M_001_007_RL/DRYER ==
  wet : Inport
  Constant1 : Constant  Value=DRY.demand.P
  Constant2 : Constant  Value=DRY.out.mfrac.H2O
  Minus : Sum  Inputs=+-
  Product : Product
  Product3 : Product
  Subsystem Reference2 : Subsystem  ReferencedSubsystem=PB2M_RltHub_002
      settings: PortSchema="{\"entries\":[{\"content\":{\"sides\":[{\"content\":{\"connectorIds\":[\"In1\",\"In2\",\"In9\",\"In3\",\"In4\",\"In5\",\"In10\",\"In11\",\"In12\",\"In13\",\"In6\",\"In7\",\"In8\"]},\"type\":\"ConnectorPlacement.EquallySpacedRectSide\",\"uuid\":\"c0facf1f-1082-4e5e-a2dc-e6e5892eaa43\"},{\"content\":{\"connectorIds\":[\"Out1\"],\"side\":\"RIGHT\"},\"type\":\"ConnectorPlacement.EquallySpacedRectSide\",\"uuid\":\"0b7dd7b0-e6ba-4d46-903a-281e0aa5a817\"},{\"content\":{\"side\":\"TOP\"},\"type\":\"ConnectorPlacement.EquallySpacedRectSide\",\"uuid\":\"7e96b7db-a9f3-428f-bb56-8b966044c518\"}]},\"type\":\"ConnectorPlacement.EquallySpacedConnector\",\"uuid\":\"c0112396-a54d-4537-ae03-3d933c26b43e\"}],\"packageUris\":[\"http://schema.mathworks.com/mf0/Connector/R2020b\"],\"version\":\"1.0\"}"
  To Workspace2 : ToWorkspace  VariableName=DRY  SampleTime=-1
  Water : Outport
  dry : Outport  Port=2
  tag scope: BM_dry=global, DRY_E=global
  wires:
  wet/1 -> Minus/1, Product/1, Subsystem Reference2/5
  Minus/1 -> [BM_dry], Subsystem Reference2/9, dry/1, Product3/1
  Product/1 -> Minus/2, Subsystem Reference2/12, Water/1
  Constant1/1 -> Product3/2
  Product3/1 -> [DRY_E], Subsystem Reference2/1
  Constant2/1 -> Product/2
  Subsystem Reference2/1 -> To Workspace2/1

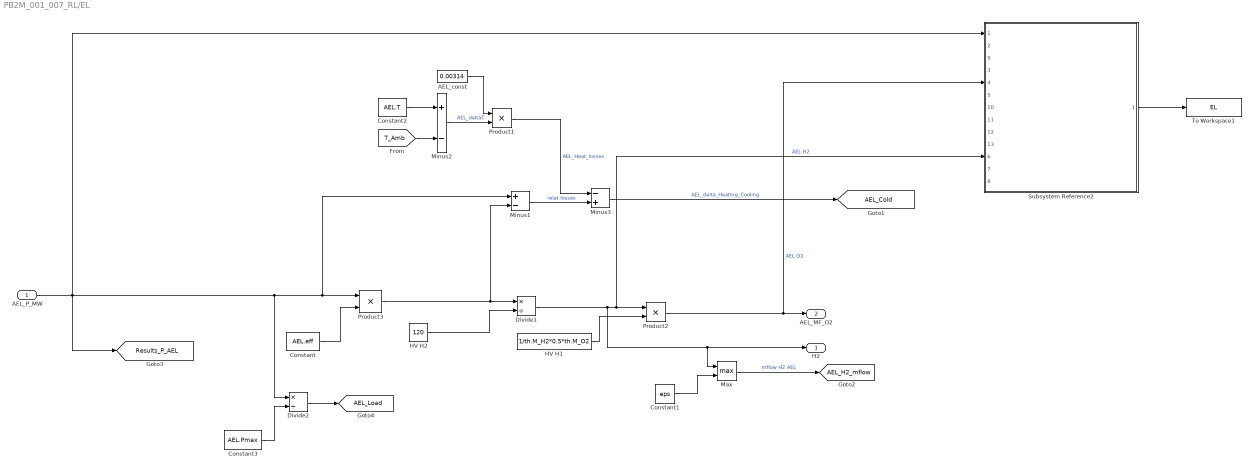
== system PB2M_001_007_RL/EL ==
  AEL_P_MW : Inport
  AEL_const : Constant  Value=0.00314
  Constant : Constant  Value=AEL.eff
  Constant1 : Constant  Value=eps
  Constant2 : Constant  Value=AEL.T
  Constant3 : Constant  Value=AEL.Pmax
  Divide1 : Product  Inputs=*/
  Divide2 : Product  Inputs=*/
  HV H1 : Constant  Value=1/th.M_H2*0.5*th.M_O2
  HV H2 : Constant  Value=120
  Max : MinMax  Function=max  Inputs=2
  Minus1 : Sum  Inputs=+-
  Minus2 : Sum  Inputs=+-
  Minus3 : Sum  Inputs=-+
  Product1 : Product
  Product2 : Product
  Product3 : Product
  Subsystem Reference2 : Subsystem  ReferencedSubsystem=PB2M_RltHub_002
      settings: PortSchema="{\"entries\":[{\"content\":{\"sides\":[{\"content\":{\"connectorIds\":[\"In1\",\"In2\",\"In9\",\"In3\",\"In4\",\"In5\",\"In10\",\"In11\",\"In12\",\"In13\",\"In6\",\"In7\",\"In8\"]},\"type\":\"ConnectorPlacement.EquallySpacedRectSide\",\"uuid\":\"c0facf1f-1082-4e5e-a2dc-e6e5892eaa43\"},{\"content\":{\"connectorIds\":[\"Out1\"],\"side\":\"RIGHT\"},\"type\":\"ConnectorPlacement.EquallySpacedRectSide\",\"uuid\":\"0b7dd7b0-e6ba-4d46-903a-281e0aa5a817\"},{\"content\":{\"side\":\"TOP\"},\"type\":\"ConnectorPlacement.EquallySpacedRectSide\",\"uuid\":\"7e96b7db-a9f3-428f-bb56-8b966044c518\"}]},\"type\":\"ConnectorPlacement.EquallySpacedConnector\",\"uuid\":\"c0112396-a54d-4537-ae03-3d933c26b43e\"}],\"packageUris\":[\"http://schema.mathworks.com/mf0/Connector/R2020b\"],\"version\":\"1.0\"}"
  To Workspace1 : ToWorkspace  VariableName=EL  SampleTime=-1
  H2 : Outport
  AEL_MF_O2 : Outport  Port=2
  tag scope: AEL_Cold=global, AEL_H2_mflow=global, AEL_Load=global, Results_P_AEL=global
  wires:
  Divide2/1 -> [AEL_Load]
  Product2/1 -> Subsystem Reference2/4, AEL_MF_O2/1  "AEL O2"
  Product3/1 -> Divide1/1, Minus1/2
  HV H2/1 -> Divide1/2
  AEL_P_MW/1 -> [Results_P_AEL], Product3/1, Minus1/1, Divide2/1, Subsystem Reference2/1
  Minus1/1 -> Minus3/2  "relat losses"
  Constant2/1 -> Minus2/1
  [T_Amb] -> Minus2/2
  Minus2/1 -> Product1/2  "AEL_deltaT"
  Minus3/1 -> [AEL_Cold]  "AEL_delta_Heating_Cooling"
  AEL_const/1 -> Product1/1
  Product1/1 -> Minus3/1  "AEL_Heat_losses"
  Divide1/1 -> Max/1, H2/1, Subsystem Reference2/6, Product2/1  "AEL H2"
  HV H1/1 -> Product2/2
  Constant1/1 -> Max/2
  Max/1 -> [AEL_H2_mflow]  "mflow H2 AEL"
  Constant3/1 -> Divide2/2
  Subsystem Reference2/1 -> To Workspace1/1
  Constant/1 -> Product3/2

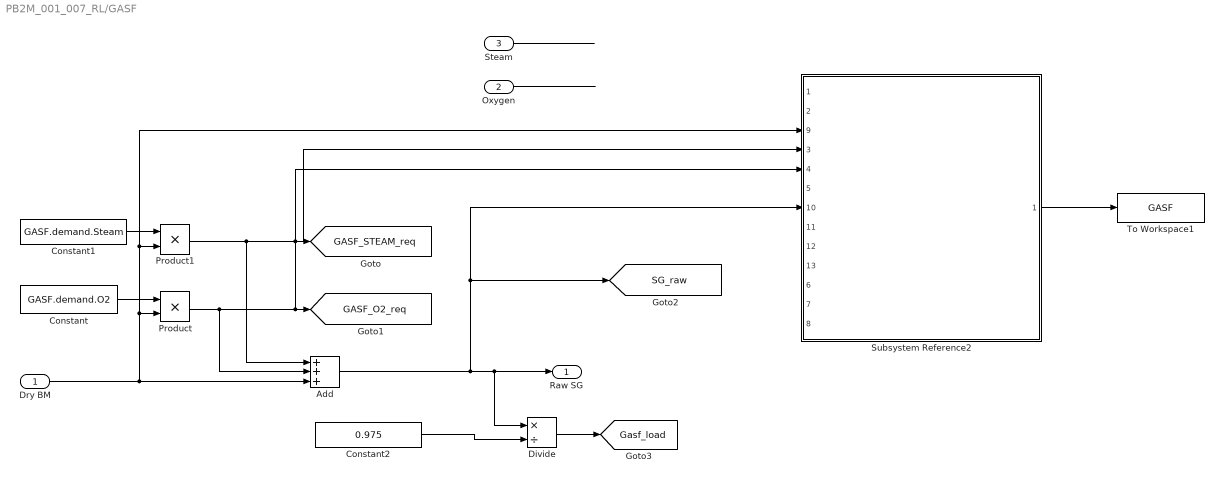
== system PB2M_001_007_RL/GASF ==
  Dry BM : Inport
  Oxygen : Inport  Port=2
  Steam : Inport  Port=3
  Add : Sum  Inputs=3
  Constant : Constant  Value=GASF.demand.O2
  Constant1 : Constant  Value=GASF.demand.Steam
  Constant2 : Constant  Value=0.975
  Divide : Product  Inputs=*/
  Product : Product
  Product1 : Product
  Subsystem Reference2 : Subsystem  ReferencedSubsystem=PB2M_RltHub_002
      settings: PortSchema="{\"entries\":[{\"content\":{\"sides\":[{\"content\":{\"connectorIds\":[\"In1\",\"In2\",\"In9\",\"In3\",\"In4\",\"In5\",\"In10\",\"In11\",\"In12\",\"In13\",\"In6\",\"In7\",\"In8\"]},\"type\":\"ConnectorPlacement.EquallySpacedRectSide\",\"uuid\":\"c0facf1f-1082-4e5e-a2dc-e6e5892eaa43\"},{\"content\":{\"connectorIds\":[\"Out1\"],\"side\":\"RIGHT\"},\"type\":\"ConnectorPlacement.EquallySpacedRectSide\",\"uuid\":\"0b7dd7b0-e6ba-4d46-903a-281e0aa5a817\"},{\"content\":{\"side\":\"TOP\"},\"type\":\"ConnectorPlacement.EquallySpacedRectSide\",\"uuid\":\"7e96b7db-a9f3-428f-bb56-8b966044c518\"}]},\"type\":\"ConnectorPlacement.EquallySpacedConnector\",\"uuid\":\"c0112396-a54d-4537-ae03-3d933c26b43e\"}],\"packageUris\":[\"http://schema.mathworks.com/mf0/Connector/R2020b\"],\"version\":\"1.0\"}"
  To Workspace1 : ToWorkspace  VariableName=GASF  SampleTime=-1
  Raw SG : Outport
  tag scope: GASF_O2_req=global, GASF_STEAM_req=global, Gasf_load=global, SG_raw=global
  wires:
  Constant/1 -> Product/1
  Dry BM/1 -> Subsystem Reference2/9, Product1/2, Product/2, Add/3
  Constant1/1 -> Product1/1
  Product1/1 -> Add/1, Subsystem Reference2/3, [GASF_STEAM_req]
  Product/1 -> Add/2, Subsystem Reference2/4, [GASF_O2_req]
  Add/1 -> Subsystem Reference2/10, [SG_raw], Divide/1, Raw SG/1
  Steam/1 -> ?
  Oxygen/1 -> ?
  Constant2/1 -> Divide/2
  Divide/1 -> [Gasf_load]
  Subsystem Reference2/1 -> To Workspace1/1

== system PB2M_001_007_RL/GRID ==
  Subsystem Reference1 : Subsystem  ReferencedSubsystem=PB2M_RltHub_002
      settings: PortSchema="{\"entries\":[{\"content\":{\"sides\":[{\"content\":{\"connectorIds\":[\"In1\",\"In2\",\"In9\",\"In10\",\"In11\",\"In12\",\"In13\",\"In3\",\"In4\",\"In5\",\"In6\",\"In7\",\"In8\"]},\"type\":\"ConnectorPlacement.EquallySpacedRectSide\",\"uuid\":\"71ace47f-78c1-4f28-9c07-d00d26defc7b\"},{\"content\":{\"connectorIds\":[\"Out1\"],\"side\":\"RIGHT\"},\"type\":\"ConnectorPlacement.EquallySpacedRectSide\",\"uuid\":\"ebbfa327-79cd-4127-8529-58e9fdc5f229\"},{\"content\":{\"side\":\"TOP\"},\"type\":\"ConnectorPlacement.EquallySpacedRectSide\",\"uuid\":\"4ee4928f-e4ee-4e39-be12-b1b382da767f\"}]},\"type\":\"ConnectorPlacement.EquallySpacedConnector\",\"uuid\":\"c0cad3a1-6b04-4e18-88e1-b09ff0fc8c60\"}],\"packageUris\":[\"http://schema.mathworks.com/mf0/Connector/R2020b\"],\"version\":\"1.0\"}"
  To Workspace : ToWorkspace  VariableName=GRID  SampleTime=-1
  OUT : Outport
  wires:
  [Power_Grid] -> OUT/1, Subsystem Reference1/1
  Subsystem Reference1/1 -> To Workspace/1

== system PB2M_001_007_RL/MS ==
  SG : Inport
  Constant1 : Constant  Value=MES.out.Purge.mfrac
  Constant2 : Constant  Value=MES.Espec
  Product1 : Product
  Product2 : Product
  Subsystem Reference2 : Subsystem  ReferencedSubsystem=PB2M_RltHub_002
      settings: PortSchema="{\"entries\":[{\"content\":{\"sides\":[{\"content\":{\"connectorIds\":[\"In1\",\"In2\",\"In9\",\"In3\",\"In4\",\"In5\",\"In10\",\"In11\",\"In12\",\"In13\",\"In6\",\"In7\",\"In8\"]},\"type\":\"ConnectorPlacement.EquallySpacedRectSide\",\"uuid\":\"c0facf1f-1082-4e5e-a2dc-e6e5892eaa43\"},{\"content\":{\"connectorIds\":[\"Out1\"],\"side\":\"RIGHT\"},\"type\":\"ConnectorPlacement.EquallySpacedRectSide\",\"uuid\":\"0b7dd7b0-e6ba-4d46-903a-281e0aa5a817\"},{\"content\":{\"side\":\"TOP\"},\"type\":\"ConnectorPlacement.EquallySpacedRectSide\",\"uuid\":\"7e96b7db-a9f3-428f-bb56-8b966044c518\"}]},\"type\":\"ConnectorPlacement.EquallySpacedConnector\",\"uuid\":\"c0112396-a54d-4537-ae03-3d933c26b43e\"}],\"packageUris\":[\"http://schema.mathworks.com/mf0/Connector/R2020b\"],\"version\":\"1.0\"}"
  To Workspace1 : ToWorkspace  VariableName=MES  SampleTime=-1
  MeOH raw : Outport
  Purge : Outport  Port=2
  tag scope: MES_E_recirc=global
  wires:
  Constant2/1 -> Product2/1
  Product2/1 -> Subsystem Reference2/1, [MES_E_recirc]
  SG/1 -> Product1/1, Subsystem Reference2/7, MeOH raw/1, Product2/2  "SG in"
  Product1/1 -> Purge/1  "purge"
  Constant1/1 -> Product1/2
  Subsystem Reference2/1 -> To Workspace1/1
  [H2_mflow_Total] -> Subsystem Reference2/6
  [SG_Reform_out] -> Subsystem Reference2/11

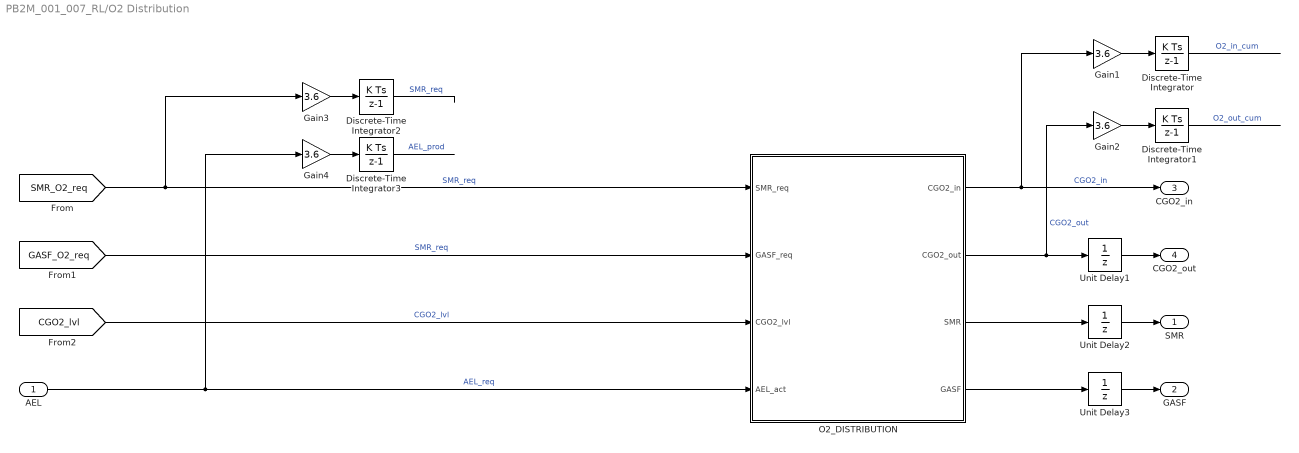
== system PB2M_001_007_RL/O2 Distribution ==
  AEL : Inport
  Discrete-Time Integrator{,1..3} (4 alike) : DiscreteIntegrator  SampleTime=-1  ICPrevOutput=DiscIntNeverNeededParam  ICPrevScaledInput=DiscIntNeverNeededParam
  Gain{1..4} (4 alike) : Gain  Gain=3.6
  O2_DISTRIBUTION : Stateflow chart  TreatAsAtomicUnit=on
      settings: PortSchema="{\"entries\":[{\"content\":{\"sides\":[{\"content\":{\"connectorIds\":[\"In1\",\"In4\",\"In3\",\"In2\"]},\"type\":\"ConnectorPlacement.EquallySpacedRectSide\",\"uuid\":\"621105b3-c3dc-4330-bdef-d993cdecb60c\"},{\"content\":{\"connectorIds\":[\"Out1\",\"Out2\",\"Out3\",\"Out4\"],\"side\":\"RIGHT\"},\"type\":\"ConnectorPlacement.EquallySpacedRectSide\",\"uuid\":\"49dd08d2-12bd-4f9c-8bf9-bd4ad8fb6d9e\"},{\"content\":{\"side\":\"TOP\"},\"type\":\"ConnectorPlacement.EquallySpacedRectSide\",\"uuid\":\"131dd091-cb90-4a7c-ba23-9028845e06c3\"}]},\"type\":\"ConnectorPlacement.EquallySpacedConnector\",\"uuid\":\"78af0694-bd8e-4e4a-a281-7245970286e6\"}],\"packageUris\":[\"http://schema.mathworks.com/mf0/Connector/R2020b\"],\"version\":\"1.0\"}"
  Unit Delay1 : UnitDelay  SampleTime=-1  HasFrameUpgradeWarning=on
  Unit Delay2 : UnitDelay  SampleTime=-1  HasFrameUpgradeWarning=on
  Unit Delay3 : UnitDelay  SampleTime=-1  HasFrameUpgradeWarning=on
  SMR : Outport
  GASF : Outport  Port=2
  CGO2_in : Outport  Port=3
  CGO2_out : Outport  Port=4
  wires:
  [SMR_O2_req] -> O2_DISTRIBUTION/1(SMR_req), Gain3/1  "SMR_req"
  O2_DISTRIBUTION/2(CGO2_out) -> Gain2/1, Unit Delay1/1  "CGO2_out"
  O2_DISTRIBUTION/3(SMR) -> Unit Delay2/1
  O2_DISTRIBUTION/1(CGO2_in) -> Gain1/1, CGO2_in/1  "CGO2_in"
  Unit Delay1/1 -> CGO2_out/1
  [CGO2_lvl] -> O2_DISTRIBUTION/3(CGO2_lvl)  "CGO2_lvl"
  Gain1/1 -> Discrete-Time Integrator/1
  Discrete-Time Integrator/1 -> ?  "O2_in_cum"
  Gain2/1 -> Discrete-Time Integrator1/1
  Discrete-Time Integrator1/1 -> ?  "O2_out_cum"
  Gain3/1 -> Discrete-Time Integrator2/1
  Discrete-Time Integrator2/1 -> ?  "SMR_req"
  Gain4/1 -> Discrete-Time Integrator3/1
  Discrete-Time Integrator3/1 -> ?  "AEL_prod"
  AEL/1 -> Gain4/1, O2_DISTRIBUTION/2(AEL_act)  "AEL_req"
  Unit Delay2/1 -> SMR/1
  Unit Delay3/1 -> GASF/1
  O2_DISTRIBUTION/4(GASF) -> Unit Delay3/1
  [GASF_O2_req] -> O2_DISTRIBUTION/4(GASF_req)  "SMR_req"

== system PB2M_001_007_RL/SG DISTR ==
  Input : Inport
  Minus : Sum  Inputs=+-
  CHP : Outport
  MSR : Outport  Port=2
  tag scope: SG_Reform_in=global, SG_chp=global
  wires:
  [CHP_SG_req] -> CHP/1, [SG_chp], Minus/2
  Input/1 -> Minus/1
  Minus/1 -> [SG_Reform_in], MSR/1

== system PB2M_001_007_RL/SG DISTR1 ==
  BIO : Inport
  E : Inport  Port=2
  Add : Sum
  Output : Outport
  tag scope: H2_mflow_Total=global, SG_mes=global
  wires:
  BIO/1 -> Add/2
  Add/1 -> [SG_mes], Output/1
  E/1 -> [H2_mflow_Total], Add/1

== system PB2M_001_007_RL/WT, PV ==
  Ambient Temperature : Lookup_n-D  NumberOfTableDimensions=1  BreakpointsForDimension1=global_time  Table=[AMB.LU.t_air]'  ExtrapMethod=Clip  InternalRulePriority=Speed  RndMeth=Simplest
  Digital Clock : DigitalClock  SampleTime=[global_ST]
  PHOTOVOLTAIC : Subsystem
  Solar Irradiance : Lookup_n-D  NumberOfTableDimensions=1  BreakpointsForDimension1=global_time  Table=[AMB.LU.G_t]'  ExtrapMethod=Clip  InternalRulePriority=Speed  RndMeth=Simplest
  Sum : Sum
  WIND TURBINE : Subsystem
  Wind Speed : Lookup_n-D  NumberOfTableDimensions=1  BreakpointsForDimension1=global_time  Table=[AMB.LU.v_wind]'  ExtrapMethod=Clip  InternalRulePriority=Speed  RndMeth=Simplest
  P_renew : Outport
  tag scope: Results_P_PV=global, Results_P_WT=global, Results_P_renew=global, T_Amb=global
  wires:
  Solar Irradiance/1 -> PHOTOVOLTAIC/1(G_t [W/m^2])  "G_t"
  Digital Clock/1 -> Wind Speed/1, Ambient Temperature/1, Solar Irradiance/1
  Ambient Temperature/1 -> [T_Amb], PHOTOVOLTAIC/2(t_amb [°C])  "t_amb"
  Wind Speed/1 -> WIND TURBINE/1(v_wind [m/s])  "v_wind"
  PHOTOVOLTAIC/1(PV_P_Out_MW) -> [Results_P_PV], Sum/1  "P_El_PV"
  Sum/1 -> P_renew/1, [Results_P_renew]  "P_El_Total"
  WIND TURBINE/1(WT_P_Out [MW]) -> [Results_P_WT], Sum/2  "P_WT"
